simulink model "eCS_Algo_Simulation_2015b_opti - original"  (R2015b)
settings: Solver=ode1  StartTime=0.0  StopTime=3  FixedStep=1/80000  RelTol=1e-3
PreLoadFcn:
  | if exist('tl_preloadfcn','file'), tl_preloadfcn(gcs,402); end
PostLoadFcn:
  | , if any(exist('dsrtsu_mdlpostloadfcn', 'file') == [2, 3, 6]), try dsrtsu_mdlpostloadfcn('Execute', bdroot); catch fprintf('Error in PostLoadFcn (dsrtsu_mdlpostloadfcn) for model "%s":\n %s\n', bdroot, lasterr); end, end,
  | if exist('tl_postloadfcn','file'), tl_postloadfcn(gcs,402); end
InitFcn:
  | Omegan=1.3024e+03;
  | xi=0.9; %0.48
  | K=0.1931;
  | K1=0.0198;
  | TauLocked=0.00255;
  | TauUnLocked=0.0042;
  | Kp=1/(2*K1);
  | Ki=Kp/((TauLocked+TauUnLocked)/2);
  | if exist('tlds_init','file'), tlds_init(gcs); end
StartFcn:
  | if exist('tlds_start','file'), tlds_start(gcs); end
StopFcn:
  | if exist('tlds_stop','file'), tlds_stop(gcs); end
model workspace (MAT data in the model file):
  au8PrevExecProfile = [0 0 0 0 0 0]
values from neighbouring files (symbols this model uses):
  AccSensor = 5    [Parameter_eCS_Algo.m]
  AlgoType = 0    [Parameter_eCS_Algo.m]
  Cxy = 1*0.017    (= 0.017)    [Acc_Init_SelV1.m]
  Cxz = 1*0.017    (= 0.017)    [Acc_Init_SelV1.m]
  Cyx = 1*0.017    (= 0.017)    [Acc_Init_SelV1.m]
  Cyz = 1*0.017    (= 0.017)    [Acc_Init_SelV1.m]
  Czx = 1*0.017    (= 0.017)    [Acc_Init_SelV1.m]
  Czy = 1*0.017    (= 0.017)    [Acc_Init_SelV1.m]
  Forced_Oscillation = 0    [Parameter_eCS_Algo.m]    (also in run_Rotation_sim.m = run)
  FreqTemperature = 10    [Acc_Init_SelV1.m]
  MaxSensorOffset = 0.3    [Acc_Init_SelV1.m]
  Mean_x_noise = 4e-3    (= 0.004)    [Acc_Init_SelV1.m]
  Mean_y_noise = 4e-3    (= 0.004)    [Acc_Init_SelV1.m]
  Mean_z_noise = 4e-3    (= 0.004)    [Acc_Init_SelV1.m]
  ODR = 8000    [Acc_Init_SelV1.m]
  offsetcorrection_on_off = 0    [Parameter_eCS_Algo.m]
  phi_pulse_rotation = 0    [Parameter_eCS_Algo.m]    (also in run_Rotation_sim.m = angle)
  pulsetype = 2    [Parameter_eCS_Algo.m]    (also in run_simulation.m = j; run_simulation_ActiveX.m = j)
  Range = 4    [Acc_Init_SelV1.m]
  sensitivity_optimisation = 0    [Parameter_eCS_Algo.m]
  TempBias = 0    [Acc_Init_SelV1.m]
  TemperatureAmp = 0    [Acc_Init_SelV1.m]
  Var_x_noise = 1.84e-9    (= 1.84e-09)    [Acc_Init_SelV1.m]
  Var_y_noise = 2.025e-09    [Acc_Init_SelV1.m]
  Var_z_noise = 1.374e-09    [Acc_Init_SelV1.m]
  w_x = 2*pi*F_x    (= 376.991118431)    [Acc_Init_SelV1.m]
  w_y = 2*pi*F_y    (= 376.991118431)    [Acc_Init_SelV1.m]
  w_z = 2*pi*F_z    (= 376.991118431)    [Acc_Init_SelV1.m]
  x_max_temp_drift = 0.061    [Acc_Init_SelV1.m]
  x_offset_enable = 0    [Acc_Init_SelV1.m]
  x_run_to_run_drift = 0.0    (= 0)    [Acc_Init_SelV1.m]
  x_temp_co_drift = 0.000    (= 0)    [Acc_Init_SelV1.m]
  Xi_x = 0.7    [Acc_Init_SelV1.m]
  Xi_y = 0.7    [Acc_Init_SelV1.m]
  Xi_z = 0.7    [Acc_Init_SelV1.m]
  y_max_temp_drift = 0.061    [Acc_Init_SelV1.m]
  y_offset_enable = 0    [Acc_Init_SelV1.m]
  y_run_to_run_drift = 0.0    (= 0)    [Acc_Init_SelV1.m]
  y_temp_co_drift = 0.000    (= 0)    [Acc_Init_SelV1.m]
  z_max_temp_drift = 0.13    [Acc_Init_SelV1.m]
  z_offset_enable = 0    [Acc_Init_SelV1.m]
  z_run_to_run_drift = 0.0    (= 0)    [Acc_Init_SelV1.m]
  z_temp_co_drift = 0.000    (= 0)    [Acc_Init_SelV1.m]
undefined symbols (not defined in the file or in its folder): ddv, DiscIntNeverNeededParam, gmw_roada_x__m_s__, gmw_roada_y__m_s__, gmw_roadtime_2kHz, KSF_50_a_x, KSF_50_a_y, KSF_50_time, KSG_30_a_x, KSG_30_a_y, KSG_30_time, Meldorf_HindenburgstraAcceleration_x__m_s_2_, Meldorf_HindenburgstraAcceleration_y__m_s_2_, Meldorf_HindenburgstraAcceleration_z__m_s_2_, Meldorf_HindenburgstraTime__s_, pulse_FF27, pulse_MPDB, pulse_ODB40, pulse_ODB64, pulse_USNCAP, pulsetime_FF27, pulsetime_MPDB, pulsetime_ODB40, pulsetime_ODB64, pulsetime_USNCAP, Rauasphalt_60_a_x, Rauasphalt_60_a_y, Rauasphalt_60_time, sigbuilder_block, VW_416_2kHza_x_2kHz, VW_416_2kHza_y_2kHz, VW_416_2kHztime_2kHz
libraries: simulink x20, tllib x16, tl_autosar_lib x12, simulink_extras x7, LIB_TF_G_12_StepControl x2, LIB_TF_G_111 x1, LIB_TF_G_112 x1
(part 1 of 9)
PreSaveFcn:
  | if exist('tl_presavefcn','file'), tl_presavefcn(gcs); end
CloseFcn:
  | if exist('tl_closefcn','file'), tl_closefcn(gcs); end
settings Model: Tag=struct('sfcnName','Subsystem_sf','subFunction','','srcSubsystem','')  DSRTSU_INTERNAL_RTI_VER=520  DSRTSU_INTERNAL_RTI_TYPE=rti1103  DSRTSU_INTERNAL_RTIFPGA=110  RTICANMMDATA=struct('GeneralSetupData',struct('modelroot','P:\ES\USER\Hinrichs\Projekte\93D48_eCS\Simulink\20200514_eCS_Simulation_package','generalsettings',struct('filesettings',struct('destfolder',struct('Name','RTICANMM_FILES','Check',1),'buildfolder',struct('Name','.','Check',1),'AbsDestfolder',struct('Name','P:\ES\USER\Hinrichs\Projekte\93D48_eCS\Simulink\20200514_eCS_Simulation_package\RTICANMM_FILES'),'AbsBuildfolder',struct('Name','P:\ES\USER\Hinrichs\Projekte\93D48_eCS\Simulink\20200514_eCS_Simulation_package'))),'options',struct('addpaths',1,'rmpaths',1,'addtrcexclusion',logical(1),'cannavigator',struct('checkmonitoring',0),'show_usrtrc',0,'use_usrtrc',0),'advanced',struct('options',[1 1 1 1 1 1 1 1 1 1 1 1 1 1 1 1 1 1 1 1 1 1 1 1 1 1 1 1 1 1 1 1 1 1 1 1 1 1 1 1 1 1 1 1 1 1 1 1 1 1 1 1 1 1 1 1 1 1 1 1 1 1 1 1 1 1 1 1 1 1 1 1 1 1 1 1 1 1 1 1 1 1 1 1 1 1 1 1 1 1 1 1 1 1 1 1 1 1 1 1]),'MPSetup',{{}},'modelname','eCS_Algo_Simulation','block','eCS_Algo_Simulation'))  DSRTSU_INTERNAL_RTIFLEXRAYCONFIG=110  TL_MAIN_DATA={'date',739018.44784596062,'advcodeopt',{'IgnoreAccessFunctionsInOwnModule';'on';'OptimizationIterationThreshold';100;'SideEffectFreeAnalysisThreshold';1000000;'ReuseStructHandling';1;'ReplaceUnrolledVectorsAndMatricesByScalars';'on';'GlobalOptimizationIterationThreshold';100;'ForceBooleanOperandsInBooleanOperations';'off'},'codegenerationmode',2}  TLRevision=402  DS_PROJECTFILE=eCS_DD.dd  Creator=heiko.hinrichs  LastModifiedBy=victor.popina
settings SolverCC: AutoInsertRateTranBlk=on
settings DataIOCC: SaveFormat=Array
settings OptimizationCC: BlockReduction=off  OptimizeBlockIOStorage=off  BufferReuse=off  GlobalBufferReuse=off  ExpressionFolding=off  ExpressionDepthLimit=2147483647  LocalBlockOutputs=off
settings DebuggingCC: UnderspecifiedInitializationDetection=Classic  MergeDetectMultiDrivingBlocksExec=none  SolverPrmCheckMsg=warning  FcnCallInpInsideContextMsg=EnableAllAsWarning  BusObjectLabelMismatch=error  AllowSymbolicDim=on  StateNameClashWarn=warning  StrictBusMsg=ErrorOnBusTreatedAsVector  NonBusSignalsTreatedAsBus=error
settings HardwareCC: ProdBitPerPointer=32  ProdLargestAtomicInteger=Integer  ProdEndianess=BigEndian  ProdWordSize=32  ProdHWDeviceType=Custom Processor->Custom  TargetHWDeviceType=Custom Processor->Custom
settings RTWCC: SystemTargetFile=rti1103.tlc  MakeCommand=make_rti  TemplateMakefile=rti1103.tmf  Description=dSPACE DS1103 Hardware Platform
settings STFCustomTargetCC: ParMdlRefBuildCompliant=on  ConcurrentExecutionCompliant=off  GeneratePreprocessorConditionals=Use local settings  CPPClassGenCompliant=off  GRTInterface=off  SystemTargetFile=rti1103.tlc
settings GRTTargetCC: CompOptLevelCompliant=off  ConcurrentExecutionCompliant=off  CombineOutputUpdateFcns=off  MatFileLogging=off  CPPClassGenCompliant=off  UseToolchainInfoCompliant=off  ExtModeMexFile=noextcomm
settings ConfigComp: CovModelRefEnable=Off

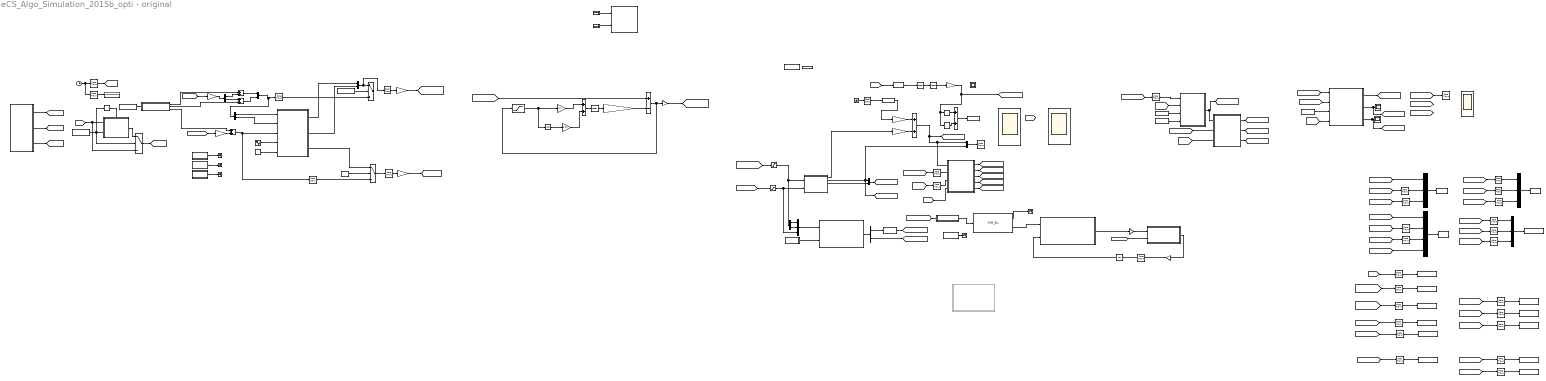
== system eCS_Algo_Simulation_2015b_opti - original ==
  note: ECS
  note: [-39.22 ; 39.22] m/s²
      | [-4 ; 4] g
  note: "retractor locked"
  note: Outputs
  note: Retractor mechanics
  note: Solenoid
  note: Offset correction
  note: Input pulses / load cases
  note: Sensor model Ziad
  note: "lever locked" (solenoid locked)
  note: "lock decision" (algo "locked")
  A_to_mA : Gain  Gain=1000
  Accelerometer : Subsystem
  Add{,1,3..5,7} (6 alike) : Sum
  Add2 : Sum  Inputs=+-
  Bus Selector1 : BusSelector  OutputSignals=b8EcsFlag,u16BallPosition
  BusCreator : BusCreator  Inputs=3
  Clock : Clock
  Compare To Constant : simulink/Logic and Bit Operations/Compare To Constant  relop=>=  const=25  OutDataTypeStr=uint8
  Compare To Constant1 : simulink/Logic and Bit Operations/Compare To Constant  relop=>=  const=50  OutDataTypeStr=uint8
  Compare To Constant4 : simulink/Logic and Bit Operations/Compare To Constant  relop=~=  const=0  OutDataTypeStr=boolean
  Constant : Constant  Value=0
  Constant2 : Constant  Value=Forced_Oscillation
  Crash signal1 : Subsystem  Tag=STV Subsys  LoadFcn=sigbuilder_block('load');  StartFcn=sigbuilder_block('start');  StopFcn=sigbuilder_block('stop');  ClipboardFcn=sigbuilder_block('clipboard');  mask(Sigbuilder block){}
      mask help: Simulink:masks:SigbuilderBlock_MD
      mask init:
      | if ~strcmp(get_param(bdroot(gcbh),'SimulationStatus'),'stopped') tuvar = sigbuilder_block('maskInit'); end
      settings: CopyFcn=sigbuilder_block('copy');  DeleteFcn=sigbuilder_block('delete');  ModelCloseFcn=sigbuilder_block('modelClose');  PreSaveFcn=sigbuilder_block('preSave');  PauseFcn=sigbuilder_block('pause');  ContinueFcn=sigbuilder_block('continue');  NameChangeFcn=sigbuilder_block('namechange');  OpenFcn=sigbuilder_block('open',[95.25 97.5 1200 576 ]);  CloseFcn=sigbuilder_block('close');
      mask Display: plot(0, 0, 100, 100,[2, 2, 32, 32, 2], [68, 8, 8, 68, 68],[32, 2], [38, 38], [32, 19, 2],[53, 60, 44], [32, 17, 17, 2],[16, 16, 31, 31]);txt = getActiveGroup(gcbh);text(2, 100, txt,'verticalAlignment', 'top');
  Crash signal3 : Subsystem  Tag=STV Subsys  LoadFcn=sigbuilder_block('load');  StartFcn=sigbuilder_block('start');  StopFcn=sigbuilder_block('stop');  ClipboardFcn=sigbuilder_block('clipboard');  mask(Sigbuilder block){}
      mask help: Simulink:masks:SigbuilderBlock_MD
      mask init:
      | if ~strcmp(get_param(bdroot(gcbh),'SimulationStatus'),'stopped') tuvar = sigbuilder_block('maskInit'); end
      settings: CopyFcn=sigbuilder_block('copy');  DeleteFcn=sigbuilder_block('delete');  ModelCloseFcn=sigbuilder_block('modelClose');  PreSaveFcn=sigbuilder_block('preSave');  PauseFcn=sigbuilder_block('pause');  ContinueFcn=sigbuilder_block('continue');  NameChangeFcn=sigbuilder_block('namechange');  OpenFcn=sigbuilder_block('open',[54 1.5 1200 540 ]);  CloseFcn=sigbuilder_block('close');
      mask Display: plot(0, 0, 100, 100,[2, 2, 32, 32, 2], [68, 8, 8, 68, 68],[32, 2], [38, 38], [32, 19, 2],[53, 60, 44], [32, 17, 17, 2],[16, 16, 31, 31]);txt = getActiveGroup(gcbh);text(2, 100, txt,'verticalAlignment', 'top');
  Data Type Conversion : DataTypeConversion
  Demux : Demux  Outputs=2
  Demux2 : Demux  Outputs=2
  Demux3 : Demux  Outputs=2
  Discrete-Time Integrator : DiscreteIntegrator  InitialConditionSetting=State (most efficient)  SampleTime=-1  ICPrevOutput=DiscIntNeverNeededParam  ICPrevScaledInput=DiscIntNeverNeededParam
  Discrete-Time Integrator1 : DiscreteIntegrator  InitialConditionSetting=State (most efficient)  SampleTime=-1  ICPrevOutput=DiscIntNeverNeededParam  ICPrevScaledInput=DiscIntNeverNeededParam
  Discrete-Time Integrator4 : DiscreteIntegrator  gainval=1  InitialConditionSetting=State (most efficient)  SampleTime=-1  LimitOutput=on  UpperSaturationLimit=0.3 * 9.81  LowerSaturationLimit=-0.3 * 9.81  ICPrevOutput=DiscIntNeverNeededParam  ICPrevScaledInput=DiscIntNeverNeededParam
  FSM : Subsystem  Tag=TargetLink Simulation Frame  Commented=on  mask(TL_SimFrame){}
      settings: CopyFcn=if exist('tl_copyfcn','file'), tl_copyfcn(gcbh); end  NameChangeFcn=if exist('tl_framenamechangefcn','file'), tl_framenamechangefcn(gcbh); end
      settings: OpenFcn=|
      | if exist('open_tlsubsystem','file')
      |    open_tlsubsystem(gcbh);
      | else
      |    tlsubsystem = ...
      |       find_system(gcb, ...
      |       'LookUnderMasks','on', ...
      |       'FollowLinks','on', ...
      |       'Tag','MIL Subsystem');
      |    open_system(tlsubsystem);
      | end
      mask Display: disp('TargetLink\nModel-\nin-the-loop\nmode')
  FSM_prrEcsAlgoFlag : Subsystem
  FSM_prrVehicleInputs : Subsystem
  G-lock Scope new : Scope  NumInputPorts=4
  Gain : Gain  Gain=AlgoType
  Gain1 : Gain  Gain=1- AlgoType
  Ground : Ground
  Input (Pulse/ Angle)1 : Subsystem
  MIL Handler : tllib/MIL Handler  data={'date',730486}
  Mux : Mux  Inputs=3
  Mux{1,3,8,10} (4 alike) : Mux  Inputs=2
  Mux2 : Mux
  Mux4 : Mux  Inputs=3
  Mux9 : Mux  Inputs=3
  Noisy : Subsystem  Tag=STV Subsys  LoadFcn=sigbuilder_block('load');  StartFcn=sigbuilder_block('start');  StopFcn=sigbuilder_block('stop');  ClipboardFcn=sigbuilder_block('clipboard');  mask(Sigbuilder block){}
      mask help: Simulink:masks:SigbuilderBlock_MD
      mask init:
      | if ~strcmp(get_param(bdroot(gcbh),'SimulationStatus'),'stopped') tuvar = sigbuilder_block('maskInit'); end
      settings: CopyFcn=sigbuilder_block('copy');  DeleteFcn=sigbuilder_block('delete');  ModelCloseFcn=sigbuilder_block('modelClose');  PreSaveFcn=sigbuilder_block('preSave');  PauseFcn=sigbuilder_block('pause');  ContinueFcn=sigbuilder_block('continue');  NameChangeFcn=sigbuilder_block('namechange');  OpenFcn=sigbuilder_block('open',[54 1.5 1200 535.5 ]);  CloseFcn=sigbuilder_block('close');
      mask Display: plot(0, 0, 100, 100,[2, 2, 32, 32, 2], [68, 8, 8, 68, 68],[32, 2], [38, 38], [32, 19, 2],[53, 60, 44], [32, 17, 17, 2],[16, 16, 31, 31]);txt = getActiveGroup(gcbh);text(2, 100, txt,'verticalAlignment', 'top');
  PWM_to_V : Gain  Gain=14/32768
  PrevSolenoidCurrent : UnitDelay  SampleTime=-1
  Pulse measured1 : RateTransition  Deterministic=off  OutPortSampleTime=1/2000
  Pulse measured2 : RateTransition
  Pulse measured3 : RateTransition  Deterministic=off  OutPortSampleTime=1/2000
  Pulse measured4 : RateTransition
  Pulse raw (g) : Gain  Gain=1/9.807
  Pulse raw (g)1 : Gain  Gain=1/9.807
  Pulse raw1 : Gain  Gain=9.807
  Pulse raw2 : Gain  Gain=9.807
  Pulse with Offsetcorr. : Gain
  Rate Transition{,1..2,4..6,9..11,15,22} (11 alike) : RateTransition
  Rate Transition{12..14,16..21} (9 alike) : RateTransition  OutPortSampleTime=1/10000
  Rate Transition{3,7,23..24,26..27,30..32} (9 alike) : RateTransition  OutPortSampleTime=1/2000
  Rate Transition25 : RateTransition  OutPortSampleTime=1/5
  S-Function Builder : S-Function  InitFcn=try, set_param(gcb,'FunctionName','FSM_SIL'), end  FunctionName=FSM_SIL  SFunctionModules=FSM_SIL_wrapper  SFunctionDeploymentMode=off  EnableBusSupport=off  mask(S-Function Builder){}
      mask help: Simulink:masks:SFunctionBuilder_MD
      mask init:
      | val = [[.9  0.75 0.75 1 1 .9 .9 1]',[1 1 0.75 0.75 .9 .9 1 .9]'];try , sys = get_param(gcb,'SfunBuilderFcnName');if isempty(sys), sys = get_param(gcb,'FunctionName'); end,catch, sys = get_param(gcb,'FunctionName'); end
      settings: CopyFcn=set_param(gcbh,'LinkStatus','none')  PreSaveFcn=try, set_param(gcb,'FunctionName','FSM_SIL'), end  OpenFcn=sfunctionwizard(gcbh)
      mask Display: plot(val(:,1),val(:,2)),disp(sys), port_label('input',1,'prrEcsAlgoFlag'), port_label('output',1,'psrSolenoidState'), port_label('output',2,'psrFsmProfile')
  SAD : Subsystem  Tag=TargetLink Simulation Frame  mask(TL_SimFrame){}
      settings: CopyFcn=if exist('tl_copyfcn','file'), tl_copyfcn(gcbh); end  NameChangeFcn=if exist('tl_framenamechangefcn','file'), tl_framenamechangefcn(gcbh); end
      settings: OpenFcn=|
      | if exist('open_tlsubsystem','file')
      |    open_tlsubsystem(gcbh);
      | else
      |    tlsubsystem = ...
      |       find_system(gcb, ...
      |       'LookUnderMasks','on', ...
      |       'FollowLinks','on', ...
      |       'Tag','MIL Subsystem');
      |    open_system(tlsubsystem);
      | end
      mask Display: disp('TargetLink\nModel-\nin-the-loop\nmode')
  Saturation : Saturate  UpperLimit=+39.3  LowerLimit=-39.3
  "Saturation acc. script, i.e.+-0,3g (max. offset of sensor after ageing)" : Saturate  UpperLimit=MaxSensorOffset * 9.807  LowerLimit=-MaxSensorOffset * 9.807
  Saturation1 : Saturate  UpperLimit=+39.22  LowerLimit=-39.22
  Scope1 : Scope  NumInputPorts=3
  Sign : Signum
  Solenoid Model : Subsystem  TreatAsAtomicUnit=on
  Subsystem : Subsystem  Tag=MIL Subsystem  Description=a  mask(MIL Subsystem){}
      settings: CopyFcn=if exist('tl_copyfcn','file'), tl_copyfcn(gcbh); end  NameChangeFcn=if exist('tl_namechangefcn','file'), tl_namechangefcn(gcbh); end  DestroyFcn=if exist('update_tl_main_dlg','file'), update_tl_main_dlg('TL_subs_display'); end
      mask Display: disp('TargetLink Subsystem')
  Switch : Switch  Criteria=u2 ~= 0
  TargetLink Main Dialog : tllib/TargetLink Main Dialog  data=[]
  Temperature : Sin  Amplitude=TemperatureAmp  Bias=TempBias  Frequency=FreqTemperature  SampleTime=0
  Terminator{,1..4} (5 alike) : Terminator
  Tilt_Lock_Scop1 : Scope  NumInputPorts=2
  To Workspace : ToWorkspace  VariableName=triggers_s  SaveFormat=Timeseries  SampleTime=-1
      settings: MaxDataPoints=1  Save2DSignal=2-D array (concatenate along first dimension)
  To Workspace1 : ToWorkspace  VariableName=pulse  SaveFormat=Timeseries  SampleTime=-1
      settings: Save2DSignal=2-D array (concatenate along first dimension)
  To Workspace10 : ToWorkspace  VariableName=time  SampleTime=-1
      settings: Save2DSignal=2-D array (concatenate along first dimension)
  To Workspace11 : ToWorkspace  VariableName=trigger_eCS_REF  SampleTime=-1
      settings: Save2DSignal=2-D array (concatenate along first dimension)
  To Workspace14 : ToWorkspace  VariableName=s_ball_REF  SampleTime=-1
      settings: Save2DSignal=2-D array (concatenate along first dimension)
  To Workspace15 : ToWorkspace  VariableName=ball_a2  SampleTime=-1
      settings: Save2DSignal=2-D array (concatenate along first dimension)
  To Workspace16 : ToWorkspace  VariableName=trigg_a2  SampleTime=-1
      settings: Save2DSignal=2-D array (concatenate along first dimension)
  To Workspace2 : ToWorkspace  VariableName=pulse_sensor_output  SaveFormat=Timeseries  SampleTime=-1
      settings: Save2DSignal=2-D array (concatenate along first dimension)
  To Workspace3 : ToWorkspace  VariableName=pulse_with_offsetcorrection  SaveFormat=Timeseries  SampleTime=-1
      settings: Save2DSignal=2-D array (concatenate along first dimension)
  To Workspace4 : ToWorkspace  VariableName=s_ball  SaveFormat=Timeseries  SampleTime=-1
      settings: Save2DSignal=2-D array (concatenate along first dimension)
  To Workspace5 : ToWorkspace  VariableName=trigger_eCS  SaveFormat=Timeseries  SampleTime=-1
      settings: Save2DSignal=2-D array (concatenate along first dimension)
  To Workspace6 : ToWorkspace  VariableName=triggers_times  SampleTime=-1
      settings: MaxDataPoints=1  Save2DSignal=2-D array (concatenate along first dimension)
  To Workspace7 : ToWorkspace  VariableName=s_rig  SaveFormat=Timeseries  SampleTime=-1
      settings: Save2DSignal=2-D array (concatenate along first dimension)
  To Workspace8 : ToWorkspace  VariableName=s_locking  SaveFormat=Timeseries  SampleTime=-1
      settings: Save2DSignal=2-D array (concatenate along first dimension)
  To Workspace9 : ToWorkspace  VariableName=triggercounts  SampleTime=-1
      settings: Save2DSignal=2-D array (concatenate along first dimension)
  Vektor_addition_Pulse1 : Fcn  Expr=sqrt( (u(1)*u(1)) + (u(2)*u(2)) )
  acc. measurement direct/via acc. sensor : Switch  Criteria=u2 > Threshold
  acc. measurement direct/via acc. sensor1 : Switch  Criteria=u2 > Threshold
  "acc. sensor type: 0=direct, 1=AD, 2=ST, 3=TDK, 4=NXP" : Constant  Value=AccSensor  VectorParams1D=off
  "acc. sensor type: 0=direct, 1=AD, 2=ST, 3=TDK, 4=NXP1" : Constant  Value=AccSensor  VectorParams1D=off
  delta-t to lock (ms) : Constant  Value=5
  delta-t to unlock (ms) : Constant  Value=7
  deviation dependent correction: 0.1/s ~10mg/s at 1m/s²deviation ~0,6°/s with saturation +-0,3g: max. 30mg/s / ~1,8°/s possible : Gain  Gain=0.1
  eCS : Subsystem  Tag=TargetLink Simulation Frame  mask(TL_SimFrame){}
      settings: CopyFcn=if exist('tl_copyfcn','file'), tl_copyfcn(gcbh); end  NameChangeFcn=if exist('tl_framenamechangefcn','file'), tl_framenamechangefcn(gcbh); end
      settings: OpenFcn=|
      | if exist('open_tlsubsystem','file')
      |    open_tlsubsystem(gcbh);
      | else
      |    tlsubsystem = ...
      |       find_system(gcb, ...
      |       'LookUnderMasks','on', ...
      |       'FollowLinks','on', ...
      |       'Tag','MIL Subsystem');
      |    open_system(tlsubsystem);
      | end
      mask Display: disp('TargetLink\nModel-\nin-the-loop\nmode')
  eCS Algo new2 : Subsystem
  eCS_prrAccelMtrPerSecSqd_stAccelMtrPerSecSqd : Subsystem
  eCS_prrEcsDiagRequest : Subsystem
  eCS_prrEcsDiagRequest_b8DiagReq1 : Subsystem
  locking distance (mm) : Constant  Value=18.13
  offset correction on/off : Gain  Gain=offsetcorrection_on_off  OutMin=[0]  OutMax=[1]
  oscilliation generator : Subsystem
  permanent correction: 0.01m/s²/s ~1mg/s ~0,06°/s : Gain  Gain=0.01
  phi-pulse-rotation (°) : Constant  Value=phi_pulse_rotation
  pulse rotation around z-axis : Subsystem
  retractor locking trigger : MATLAB Function  TreatAsAtomicUnit=on
  s-locking retractor (mm) : Scope
  s-rig (mm) new : Scope
  s-rig-trigger new : DataTypeConversion
  s-rig-trigger new1 : DataTypeConversion
  s_rig in mm : Gain  Gain=1000
  solenoid time delay : MATLAB Function  TreatAsAtomicUnit=on
  time (0.2s-steps) : Display
  "trigger travels, times and counts" : MATLAB Function  TreatAsAtomicUnit=on
  "trigger travels, times and counts1" : MATLAB Function  TreatAsAtomicUnit=on
  triggertime_retractor (ms) : Scope
  wires:
  Discrete-Time Integrator1/1 -> s_rig in mm/1
  Discrete-Time Integrator/1 -> Discrete-Time Integrator1/1
  Add4/1 -> "trigger travels, times and counts"/1(trigger), Mux3/1, [trigger_eCS]
  s_rig in mm/1 -> [s], Compare To Constant/1, Compare To Constant1/1
  Compare To Constant/1 -> Add/2
  Compare To Constant1/1 -> Add/1
  Add/1 -> s-rig-trigger new/1
  Mux3/1 -> Rate Transition4/1
  "Saturation acc. script, i.e.+-0,3g (max. offset of sensor after ageing)"/1 -> Sign/1, deviation dependent correction: 0.1/s ~10mg/s at 1m/s²deviation ~0,6°/s with saturation +-0,3g: max. 30mg/s / ~1,8°/s possible/1
  Sign/1 -> permanent correction: 0.01m/s²/s ~1mg/s ~0,06°/s/1
  offset correction on/off/1 -> Add2/2
  Discrete-Time Integrator4/1 -> offset correction on/off/1
  Add3/1 -> Discrete-Time Integrator4/1
  deviation dependent correction: 0.1/s ~10mg/s at 1m/s²deviation ~0,6°/s with saturation +-0,3g: max. 30mg/s / ~1,8°/s possible/1 -> Add3/1
  permanent correction: 0.01m/s²/s ~1mg/s ~0,06°/s/1 -> Add3/2
  Add2/1 -> Pulse with Offsetcorr./1, "Saturation acc. script, i.e.+-0,3g (max. offset of sensor after ageing)"/1
  Clock/1 -> Rate Transition25/1, Rate Transition2/1
  [time] -> solenoid time delay/2(time)
  [trigger_eCS] -> Rate Transition/1
  solenoid time delay/1(trigger_out) -> "trigger travels, times and counts1"/1(trigger), [locking_solenoid]
  [trigger_eCS] -> Rate Transition1/1
  Temperature/1 -> Accelerometer/4(Temperature)
  Constant/1 -> Accelerometer/5(Max temp. drift)
  Accelerometer/2(Out Y) -> Mux8/2  "sensor_ay"
  Accelerometer/1(Out X) -> Mux8/1  "sensor_ax"
  Demux2/2 -> Accelerometer/2(In Y)
  Crash signal1/1(Signal 1) -> Terminator/1
  Demux2/1 -> Accelerometer/1(In X)
  Pulse with Offsetcorr./1 -> [Pulse_with_offsetcorrection]
  locking distance (mm)/1 -> retractor locking trigger/3(s_mech_locking)
  [time] -> retractor locking trigger/4(time)
  [s] -> retractor locking trigger/2(s)
  [locking_solenoid] -> retractor locking trigger/1(trigger_solenoid)
  retractor locking trigger/1(trigger_retractor) -> [locking_retractor]
  retractor locking trigger/2(triggertime_retractor) -> [triggertime_retractor], triggertime_retractor (ms)/1
  retractor locking trigger/3(s_locking) -> [s_locking_retractor], s-locking retractor (mm)/1
  [Pulse] -> Vektor_addition_Pulse1/1
  Vektor_addition_Pulse1/1 -> Discrete-Time Integrator/1
  [Pulse_no_offsetcorrection] -> Add2/1
  Noisy/1(Signal 1) -> Terminator2/1
  Crash signal3/1(Signal 1) -> Terminator3/1
  Rate Transition/1 -> solenoid time delay/1(trigger)
  Mux/1 -> To Workspace/1
  Rate Transition2/1 -> [time]
  [time] -> Rate Transition5/1
  Rate Transition5/1 -> "trigger travels, times and counts"/3(time)
  "trigger travels, times and counts"/2(triggertime) -> [triggertime_eCS]
  [s_locking_retractor] -> Rate Transition6/1
  Rate Transition6/1 -> Mux/3
  [triggertime_eCS] -> Mux2/1
  [triggertime_solenoid] -> Rate Transition9/1
  Rate Transition9/1 -> Mux2/2
  [triggertime_retractor] -> Rate Transition10/1
  Rate Transition10/1 -> Mux2/3
  "trigger travels, times and counts"/1(s_locking) -> [s_locking_eCS]
  [s] -> Rate Transition11/1
  Rate Transition11/1 -> "trigger travels, times and counts"/2(s)
  [s_locking_eCS] -> Mux/1
  [s] -> "trigger travels, times and counts1"/2(s)
  [time] -> "trigger travels, times and counts1"/3(time)
  "trigger travels, times and counts1"/2(triggertime) -> [triggertime_solenoid]
  "trigger travels, times and counts1"/1(s_locking) -> [s_locking_solenoid]
  [s_locking_solenoid] -> Rate Transition15/1
  Rate Transition15/1 -> Mux/2
  delta-t to unlock (ms)/1 -> solenoid time delay/4(dt_to_unlock)
  delta-t to lock (ms)/1 -> solenoid time delay/3(dt_to_lock)
  Mux8/1 -> Pulse measured1/1, acc. measurement direct/via acc. sensor/1
  "acc. sensor type: 0=direct, 1=AD, 2=ST, 3=TDK, 4=NXP"/1 -> acc. measurement direct/via acc. sensor/2
  Pulse measured2/1 -> acc. measurement direct/via acc. sensor/3
  [Pulse] -> Rate Transition16/1
  Rate Transition16/1 -> To Workspace1/1
  Rate Transition17/1 -> To Workspace2/1
  [Pulse_no_offsetcorrection] -> Rate Transition17/1
  Rate Transition18/1 -> To Workspace3/1
  [Pulse_with_offsetcorrection] -> Rate Transition18/1
  Rate Transition19/1 -> To Workspace4/1
  [s_ball] -> Rate Transition19/1
  Rate Transition20/1 -> To Workspace5/1
  Mux2/1 -> To Workspace6/1
  Rate Transition13/1 -> To Workspace7/1
  [s] -> Rate Transition13/1
  Rate Transition12/1 -> Mux4/2
  [s_locking_solenoid] -> Rate Transition12/1
  [s_locking_eCS] -> Rate Transition21/1
  Rate Transition14/1 -> Mux4/3
  [s_locking_retractor] -> Rate Transition14/1
  Mux4/1 -> To Workspace8/1
  Rate Transition21/1 -> Mux4/1
  [Pulse_with_offsetcorrection] -> Saturation/1
  Rate Transition22/1 -> s-rig-trigger new1/1
  s-rig-trigger new1/1 -> Gain/1
  Gain/1 -> Add4/1
  Gain1/1 -> Add4/2
  "trigger travels, times and counts"/3(triggercounts) -> [triggercounts_eCS]
  "trigger travels, times and counts1"/3(triggercounts) -> [triggercounts_solenoid]
  [triggercounts_solenoid] -> Rate Transition24/1
  [triggercounts_eCS] -> Rate Transition23/1
  Rate Transition23/1 -> Mux9/1
  Rate Transition24/1 -> Mux9/2
  Rate Transition25/1 -> time (0.2s-steps)/1
  [time] -> Rate Transition26/1
  Rate Transition26/1 -> To Workspace10/1
  [trigger_eCS] -> Rate Transition20/1
  Rate Transition27/1 -> To Workspace11/1
  Rate Transition30/1 -> To Workspace14/1
  [trigger_eCS] -> Rate Transition27/1
  [s_ball_only] -> Rate Transition30/1
  Saturation/1 -> Demux/1, eCS Algo new2/1(Pulse X,Y)
  [Trigg_a2] -> Rate Transition32/1
  [Ball_a2] -> Rate Transition31/1
  Rate Transition31/1 -> To Workspace15/1
  Rate Transition32/1 -> To Workspace16/1
  Pulse measured1/1 -> Pulse raw1/1
  Pulse raw1/1 -> [Pulse_no_offsetcorrection]
  [Pulse_rotated] -> Pulse raw (g)/1
  Input (Pulse/ Angle)1/1("Pulse_profile ") -> [Pulse]  "pulse X,Y in m/s²"
  Input (Pulse/ Angle)1/3(angle in °) -> [angle]
  [Pulse] -> Switch/3, pulse rotation around z-axis/1(pulse in m/s²)
  phi-pulse-rotation (°)/1 -> Switch/2, Compare To Constant4/1, pulse rotation around z-axis/2(rotation angle)
  Compare To Constant4/1 -> pulse rotation around z-axis/Enable
  pulse rotation around z-axis/1(pulse rotated in m/s²) -> Switch/1
  Input (Pulse/ Angle)1/2(Pulse z-axis) -> [Pulse_z_axis]  "pulse Z in m/s²"
  [Pulse_z_axis] -> Pulse raw (g)1/1
  Accelerometer/3(Out Z) -> acc. measurement direct/via acc. sensor1/1  "sensor_az"
  Pulse measured3/1 -> Pulse raw2/1
  "acc. sensor type: 0=direct, 1=AD, 2=ST, 3=TDK, 4=NXP1"/1 -> acc. measurement direct/via acc. sensor1/2
  Pulse raw2/1 -> [Pulse_z_axis_sensor]
  Pulse measured4/1 -> acc. measurement direct/via acc. sensor1/3
  eCS Algo new2/2(s_ball) -> [s_ball_only], Mux10/1, Mux3/2  "pBall_Simulink"
  eCS Algo new2/1(Trigger eCS) -> Gain1/1
  eCS Algo new2/3(s_ball_x- + y-components) -> Mux10/2
  [Pulse_z_axis_sensor] -> Saturation1/1
  Mux10/1 -> [s_ball]
  [Trigg_a2] -> "trigger travels, times and counts"/4(eCSTrigger)
  "trigger travels, times and counts"/4(triggerCountsTL) -> [triggercounts_TL]
  Mux9/1 -> To Workspace9/1
  [triggercounts_TL] -> Rate Transition3/1
  Rate Transition3/1 -> Mux9/3
  "trigger travels, times and counts"/5(triggerTimeTL) -> [triggerTme_TL]
  [triggerTme_TL] -> Mux2/4
  acc. measurement direct/via acc. sensor1/1 -> Pulse measured3/1
  Switch/1 -> [Pulse_rotated]
  Mux1/1 -> Demux2/1, Pulse measured2/1
  Pulse raw (g)/1 -> Demux3/1
  Pulse raw (g)1/1 -> Add5/2
  Add5/1 -> Accelerometer/3(In Z), Pulse measured4/1
  Demux3/2 -> Add7/1
  Demux3/1 -> Add1/2
  Add1/1 -> Mux1/1
  Add7/1 -> Mux1/2
  Constant2/1 -> oscilliation generator/1(bOscillationReq)
  oscilliation generator/1(Oscillation_ax) -> Add1/1
  oscilliation generator/2(Oscillation_ay) -> Add7/2
  oscilliation generator/3(Oscillation_az) -> Add5/1
  FSM_prrEcsAlgoFlag/1(isrEcsAlgoOutputs) -> S-Function Builder/1
  [Trigg_a2] -> FSM_prrEcsAlgoFlag/1(EcsFlag)
  S-Function Builder/2 -> SAD/1(prrFsmProfile)
  Ground/1 -> Rate Transition22/1
  Rate Transition7/1 -> PrevSolenoidCurrent/1
  PWM_to_V/1 -> Solenoid Model/1(SolenoidVoltage)
  A_to_mA/1 -> Rate Transition7/1
  [Trigg_a2] -> Solenoid Model/2(eCS_Trigger)
  PrevSolenoidCurrent/1 -> SAD/2(sim_au16Current)
  SAD/1(pseSolenoidPWM) -> PWM_to_V/1
  eCS_prrEcsDiagRequest_b8DiagReq1/1(b8DiagReq) -> eCS/2(prrEcsDiagRequest)
  Demux/1 -> BusCreator/1  "s16Ax"
  Demux/2 -> BusCreator/2  "s16Ay"
  Saturation1/1 -> eCS Algo new2/2(Pulse Z), BusCreator/3  "s16Az"
  BusCreator/1 -> eCS/1(prrAccelMtrPerSecSqd)  "stAccelMtrPerSecSqd"
  eCS/1(psrEcsAlgoData) -> Bus Selector1/1
  Bus Selector1/1 -> Data Type Conversion/1  "<b8EcsFlag>"
  Bus Selector1/2 -> [Ball_a2]  "<u16BallPosition>"
  Data Type Conversion/1 -> [Trigg_a2]
  Solenoid Model/1(SolenoidCurrent) -> A_to_mA/1
  S-Function Builder/1 -> Terminator4/1
  FSM_prrVehicleInputs/1(isrVehicleInputs) -> Terminator1/1
  eCS_prrAccelMtrPerSecSqd_stAccelMtrPerSecSqd/1(stAccelMtrPerSecSqd) -> Subsystem/1(prrAccelMtrPerSecSqd)
  eCS_prrEcsDiagRequest/1(isrEcsDiagRequest) -> Subsystem/2(prrEcsDiagRequest)

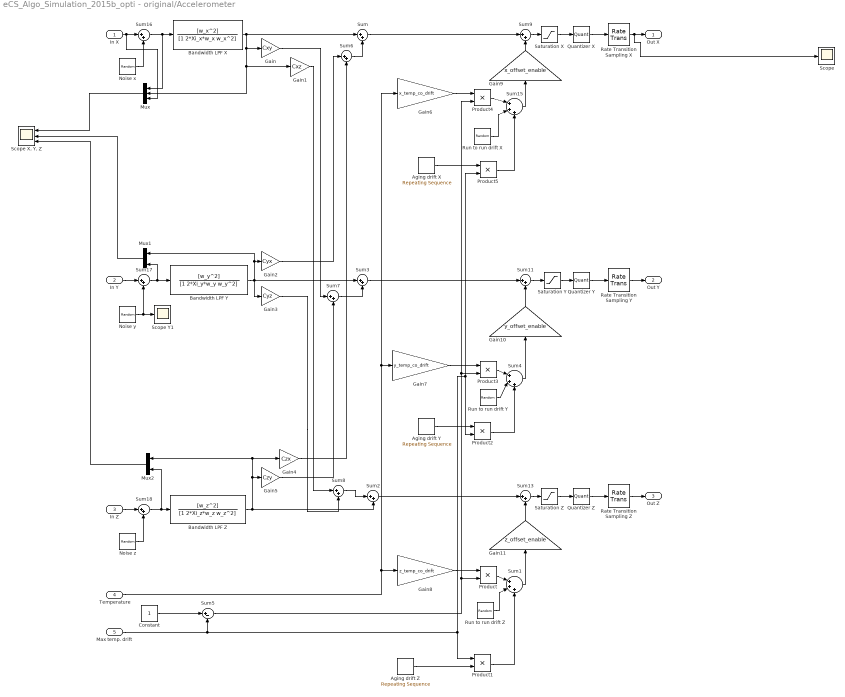
== system eCS_Algo_Simulation_2015b_opti - original/Accelerometer ==
  In X : Inport
  In Y : Inport  Port=2
  In Z : Inport  Port=3
  Temperature : Inport  Port=4
  Max temp. drift : Inport  Port=5
  Aging drift X : simulink/Sources/Repeating Sequence  rep_seq_t=[0 0.1]  rep_seq_y=[0 x_max_temp_drift]
  Aging drift Y : simulink/Sources/Repeating Sequence  rep_seq_t=[0 1000]  rep_seq_y=[0 y_max_temp_drift]
  Aging drift Z : simulink/Sources/Repeating Sequence  rep_seq_t=[0 0.001]  rep_seq_y=[0 z_max_temp_drift]
  Bandwidth LPF X : TransferFcn  Numerator=[w_x^2]  Denominator=[1 2*Xi_x*w_x w_x^2]
  Bandwidth LPF Y : TransferFcn  Numerator=[w_y^2]  Denominator=[1 2*Xi_y*w_y w_y^2]
  Bandwidth LPF Z : TransferFcn  Numerator=[w_z^2]  Denominator=[1 2*Xi_z*w_z w_z^2]
  Constant : Constant
  Gain : Gain  Gain=Cxy
  Gain1 : Gain  Gain=Cxz
  Gain10 : Gain  Gain=y_offset_enable
  Gain11 : Gain  Gain=z_offset_enable
  Gain2 : Gain  Gain=Cyx
  Gain3 : Gain  Gain=Cyz
  Gain4 : Gain  Gain=Czx
  Gain5 : Gain  Gain=Czy
  Gain6 : Gain  Gain=x_temp_co_drift
  Gain7 : Gain  Gain=y_temp_co_drift
  Gain8 : Gain  Gain=z_temp_co_drift
  Gain9 : Gain  Gain=x_offset_enable
  Mux : Mux  Inputs=3
  Mux1 : Mux  Inputs=2
  Mux2 : Mux  Inputs=2
  Noise x : RandomNumber  Mean=Mean_x_noise  Variance=Var_x_noise
  Noise y : RandomNumber  Mean=Mean_y_noise  Variance=Var_y_noise
  Noise z : RandomNumber  Mean=Mean_z_noise  Variance=Var_z_noise
  Product{,1..5} (6 alike) : Product  RndMeth=Zero
  Quantizer X : Quantizer  QuantizationInterval=Resolution
  Quantizer Y : Quantizer  QuantizationInterval=Resolution
  Quantizer Z : Quantizer  QuantizationInterval=Resolution
  Rate Transition Sampling X : RateTransition  OutPortSampleTime=1/ODR
  Rate Transition Sampling Y : RateTransition  OutPortSampleTime=1/ODR
  Rate Transition Sampling Z : RateTransition  OutPortSampleTime=1/ODR
  Run to run drift X : RandomNumber  Mean=x_run_to_run_drift  Variance=0.00001
  Run to run drift Y : RandomNumber  Mean=y_run_to_run_drift  Variance=0.00001
  Run to run drift Z : RandomNumber  Mean=z_run_to_run_drift  Variance=0.00001
  Saturation X : Saturate  UpperLimit=Range  LowerLimit=-Range
  Saturation Y : Saturate  UpperLimit=Range  LowerLimit=-Range
  Saturation Z : Saturate  UpperLimit=Range  LowerLimit=-Range
  Scope : Scope
  "Scope X, Y, Z" : Scope  NumInputPorts=3
  Scope Y1 : Scope
  Sum{,2..3,6..9,11,13,16..18} (12 alike) : Sum  Inputs=|++
  Sum1 : Sum  Inputs=|+++
  Sum15 : Sum  Inputs=|+++
  Sum4 : Sum  Inputs=|+++
  Sum5 : Sum  Inputs=|+-
  Out X : Outport
  Out Y : Outport  Port=2
  Out Z : Outport  Port=3
  wires:
  Run to run drift Z/1 -> Sum1/2
  Sum4/1 -> Gain10/1
  Run to run drift Y/1 -> Sum4/2
  Sum1/1 -> Gain11/1
  Bandwidth LPF Y/1 -> Gain3/1, Sum3/1, Mux1/1, Gain2/1
  Sum6/1 -> Sum/2
  Gain4/1 -> Sum6/2
  Bandwidth LPF Z/1 -> Mux2/1, Gain4/1, Gain5/1, Sum2/2
  Quantizer X/1 -> Rate Transition Sampling X/1
  Saturation Y/1 -> Quantizer Y/1
  Quantizer Z/1 -> Rate Transition Sampling Z/1
  Sum7/1 -> Sum3/2
  Gain5/1 -> Sum7/2
  Saturation X/1 -> Quantizer X/1
  Sum/1 -> Sum9/1
  Sum9/1 -> Saturation X/1
  Gain2/1 -> Sum6/1
  Sum3/1 -> Sum11/1
  Sum2/1 -> Sum13/1
  Sum13/1 -> Saturation Z/1
  Gain1/1 -> Sum8/1
  Run to run drift X/1 -> Sum15/2
  Gain3/1 -> Sum8/2
  Sum15/1 -> Gain9/1
  Sum11/1 -> Saturation Y/1
  In X/1 -> Mux/3, Sum16/1
  Sum16/1 -> Mux/1, Bandwidth LPF X/1
  Bandwidth LPF X/1 -> Mux/2, Gain1/1, Gain/1, Sum/1
  Gain/1 -> Sum7/1
  Quantizer Y/1 -> Rate Transition Sampling Y/1
  Saturation Z/1 -> Quantizer Z/1
  Noise z/1 -> Sum18/2
  Rate Transition Sampling Y/1 -> Out Y/1
  Sum17/1 -> Mux1/2, Bandwidth LPF Y/1
  Sum18/1 -> Bandwidth LPF Z/1, Mux2/2
  In Z/1 -> Sum18/1
  In Y/1 -> Sum17/1
  Rate Transition Sampling X/1 -> Scope/1, Out X/1
  Noise y/1 -> Scope Y1/1, Sum17/2
  Rate Transition Sampling Z/1 -> Out Z/1
  Noise x/1 -> Sum16/2
  Mux2/1 -> "Scope X, Y, Z"/3
  Temperature/1 -> Gain6/1, Gain7/1, Gain8/1
  Mux/1 -> "Scope X, Y, Z"/1
  Constant/1 -> Sum5/1
  Max temp. drift/1 -> Product2/2, Product5/2, Product1/1, Sum5/2
  Gain8/1 -> Product/1
  Product/1 -> Sum1/1
  Sum5/1 -> Product4/2, Product3/2, Product/2
  Product1/1 -> Sum1/3
  Aging drift Z/1 -> Product1/2
  Gain7/1 -> Product3/1
  Product3/1 -> Sum4/1
  Gain6/1 -> Product4/1
  Product4/1 -> Sum15/1
  Aging drift X/1 -> Product5/1
  Product5/1 -> Sum15/3
  Product2/1 -> Sum4/3
  Aging drift Y/1 -> Product2/1
  Sum8/1 -> Sum2/1
  Mux1/1 -> "Scope X, Y, Z"/2
  Gain9/1 -> Sum9/2
  Gain10/1 -> Sum11/2
  Gain11/1 -> Sum13/2

== system eCS_Algo_Simulation_2015b_opti - original/Crash signal1 ==
  Demux : Demux  Tag=STV Demux  Outputs=1
  FromWs : FromWorkspace  Tag=STV FromWs  VariableName=tuvar  SampleTime=0
      SigBuilderData=|
      | common.afterFinalStr = 'Extrapolate'
      | common.sampleTime = 0
      | dataSet.timeRange = [0 0.01]
      | dataSet.name = 'Group 1'
      | sbobj.Groups.Name = 'Group 1'
      | sbobj.Groups.Signals.Name = 'Signal 1'
      | sbobj.Groups.Signals.XData = [0 0.0005 0.001 0.001 0.0015 0.002 0.0025 0.00299 0.00299 0.0035 0.004 0.004 0.0045 0.0045 0.005 0.005 0.0055 0.0055 0.006 0.006 0.0065 0.007 0.007 0.0075 0.008 0.008 0.0085 0.009 0.0095 0.0095 0.01]
      | sbobj.Groups.Signals.YData = [0 2 2 1.99 2 2 2 2 0 0 0.015 0.02 0.005 0 2 2.005 3.96 3.98 6.04 6.03 6.02 6.04 6.06 6 5.98 0 -0.02 6 -0.02 0 0]
      | sbobj.Groups.TimeRange = [0 0.01]
  Signal 1 : Outport  Tag=STV Outport
  wires:
  Demux/1 -> Signal 1/1
  FromWs/1 -> Demux/1

== system eCS_Algo_Simulation_2015b_opti - original/Crash signal3 ==
  Demux : Demux  Tag=STV Demux  Outputs=1
  FromWs : FromWorkspace  Tag=STV FromWs  VariableName=tuvar  SampleTime=0
      SigBuilderData=|
      | common.afterFinalStr = 'Extrapolate'
      | common.sampleTime = 0
      | dataSet.timeRange = [0 0.01]
      | dataSet.name = 'Group 1'
      | sbobj.Groups.Name = 'Group 1'
      | sbobj.Groups.Signals.Name = 'Signal 1'
      | sbobj.Groups.Signals.XData = [0 0.0005 0.001 0.001 0.0015 0.002 0.0025 0.003 0.003 0.0035 0.004 0.004 0.0045 0.0045 0.005 0.005 0.0055 0.0055 0.006 0.006 0.0065 0.007 0.007 0.0075 0.008 0.008 0.0085 0.009 0.0095 0.0095 0.01]
      | sbobj.Groups.Signals.YData = [0 2 2 1.99 2 2 2 2 0 0 0.015 0.02 0.005 0 2 2.005 3.96 3.98 6.04 6.03 6.02 6.04 6.06 6 5.98 0 -0.02 6 -0.02 0 0]
      | sbobj.Groups.TimeRange = [0 0.01]
  Signal 1 : Outport  Tag=STV Outport
  wires:
  Demux/1 -> Signal 1/1
  FromWs/1 -> Demux/1

== system eCS_Algo_Simulation_2015b_opti - original/FSM ==
  prrEcsAlgoFlag : Inport
  Subsystem : Subsystem  Tag=struct('sfcnName','FSM_sf','subFunction','','srcSubsystem','')  mask(TL_Enable){}
      settings: OpenFcn=warndlg(get_param(gcb,'MaskHelp'),'Serious Warning');
      mask Help: This subsystem keeps the TargetLink subsystem (subsystem with TargetLink blocks for production code generation), and is needed for the TargetLink simulation frame to work properly. DO NOT DELETE OR MODIFY IT!
  psrSolenoidState : Outport
  psrFsmProfile : Outport  Port=2
  wires:
  prrEcsAlgoFlag/1 -> Subsystem/1(prrEcsAlgoFlag)
  Subsystem/1(psrSolenoidState) -> psrSolenoidState/1
  Subsystem/2(psrFsmProfile) -> psrFsmProfile/1

== system eCS_Algo_Simulation_2015b_opti - original/FSM_prrEcsAlgoFlag ==
  EcsFlag : Inport
  BusCreator : BusCreator  Inputs=2
  Const1 : Constant  Value=0
  isrEcsAlgoOutputs : Outport
  wires:
  EcsFlag/1 -> BusCreator/1  "b8EcsFlag"
  Const1/1 -> BusCreator/2  "u16BallPosition"
  BusCreator/1 -> isrEcsAlgoOutputs/1  "isrEcsAlgoOutputs"

== system eCS_Algo_Simulation_2015b_opti - original/FSM_prrVehicleInputs ==
  BusCreator : BusCreator  Inputs=2
  Const1 : Constant  Value=3
  Pulse measured1 : RateTransition  Deterministic=off  OutPortSampleTime=1/2000
  Ramp : simulink/Sources/Ramp  slope=1000  start=0  X0=0
  Scope : Scope
  isrVehicleInputs : Outport
  wires:
  Ramp/1 -> BusCreator/1, Scope/1  "u16Vx"
  Const1/1 -> BusCreator/2  "u8BuckleState"
  BusCreator/1 -> Pulse measured1/1  "isrVehicleInputs"
  Pulse measured1/1 -> isrVehicleInputs/1

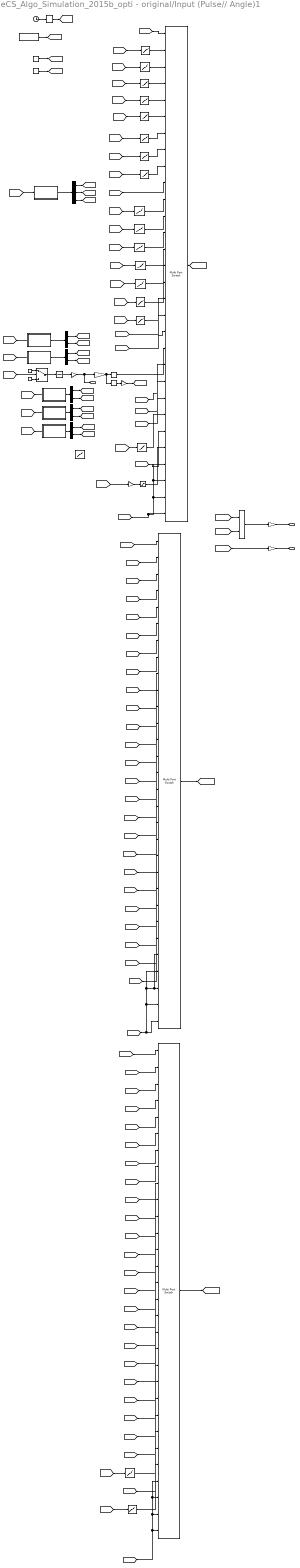
== system eCS_Algo_Simulation_2015b_opti - original/Input (Pulse// Angle)1 ==
  note: pulse tables must begin and end with 0 !!!!!!!
  -1.0 : Constant  Value=-1
  BMW QV72003-3 no-fire lower : Lookup_n-D  NumberOfTableDimensions=1  BreakpointsForDimension1=[-0.011 0.00 0.020 0.045 0.059]  Table=[0 0 11.0 11.0 0]  ExtrapMethod=Clip  UseLastTableValue=on  InternalRulePriority=Speed  RndMeth=Simplest  InputSameDT=on
  BMW QV72003-3 no-fire upper : Lookup_n-D  NumberOfTableDimensions=1  BreakpointsForDimension1=[0 0.027 0.059 0.085]  Table=[0 16.2 16.2 0]  ExtrapMethod=Clip  UseLastTableValue=on  InternalRulePriority=Speed  RndMeth=Simplest  InputSameDT=on
  Clock : Clock
  Demux1 : Demux  Outputs=3
  Demux{2..6} (5 alike) : Demux  Outputs=2
  Discrete-Time Integrator4 : DiscreteIntegrator  gainval=1  InitialConditionSetting=State (most efficient)  SampleTime=-1  UpperSaturationLimit=0.3 * 9.81  LowerSaturationLimit=-0.3 * 9.81  ICPrevOutput=DiscIntNeverNeededParam  ICPrevScaledInput=DiscIntNeverNeededParam
  Gain : Gain  Gain=-1
  Multiport Switch1 : MultiPortSwitch  Inputs=28  DataPortForDefault=Additional data port
  Multiport Switch2 : MultiPortSwitch  Inputs=28  DataPortForDefault=Additional data port
  Multiport Switch3 : MultiPortSwitch  Inputs=28  DataPortForDefault=Additional data port
  Mux1 : Mux  Inputs=2
  Puls_BMW_KSF_50 : Subsystem
  Puls_BMW_KSG_30 : Subsystem
  "Puls_BMW_Rauasphalt_60 " : Subsystem
  Puls_GWM_road_C.Morgan : Subsystem
  Puls_Kopfsteinpflaster Meldorf Hindenburgstrasse : Subsystem
  Puls_VW416_Atlas_C.Morgan : Subsystem
  Pulse table FF27 (g) : Lookup  InputValues=pulsetime_FF27  Table=pulse_FF27  LookUpMeth=Interpolation-Use End Values
  Pulse table MPDB (g) : Lookup  InputValues=pulsetime_MPDB  Table=pulse_MPDB  LookUpMeth=Interpolation-Use End Values
  Pulse table ODB40 (g) : Lookup  InputValues=pulsetime_ODB40  Table=pulse_ODB40  LookUpMeth=Interpolation-Use End Values
  Pulse table ODB64 (g) : Lookup  InputValues=pulsetime_ODB64  Table=pulse_ODB64  LookUpMeth=Interpolation-Use End Values
  Pulse table USNCAP (g) : Lookup  InputValues=pulsetime_USNCAP  Table=pulse_USNCAP  LookUpMeth=Interpolation-Use End Values
  Rate Transition : RateTransition
  Saturation : Saturate  UpperLimit=5  LowerLimit=0
  Sin1 : Trigonometry  Operator=cos
  Sin2 : Trigonometry
  Switch : Switch  Criteria=u2 > Threshold  Threshold=36
  crash angle in rad : Gain  Gain=2*pi/360
  g in m/s² : Gain  Gain=9.807
  g in m/s²1 : Gain  Gain=9.807
  "g-lock \" must lock\" - 6g/s - 0.45g" : Lookup_n-D  NumberOfTableDimensions=1  BreakpointsForDimension1=[0 0.075 0.3 0.4]  Table=[0 0.45 0.45 0]  ExtrapMethod=Clip  UseLastTableValue=on  InternalRulePriority=Speed  RndMeth=Simplest  InputSameDT=on
  "g-lock \" no lock\" - 6g/s - 0.3g" : Lookup_n-D  NumberOfTableDimensions=1  BreakpointsForDimension1=[0 0.050 0.5 0.6]  Table=[0 0.3 0.3 0]  ExtrapMethod=Clip  UseLastTableValue=on  InternalRulePriority=Speed  RndMeth=Simplest  InputSameDT=on
  g-lock Crash - 2000g/s - 30g : Lookup_n-D  NumberOfTableDimensions=1  BreakpointsForDimension1=[0 0.015 0.055 0.08]  Table=[0 30 30 0]  ExtrapMethod=Clip  UseLastTableValue=on  InternalRulePriority=Speed  RndMeth=Simplest  InputSameDT=on
  g-lock ECE - 150g/s - 0.45g : Lookup_n-D  NumberOfTableDimensions=1  BreakpointsForDimension1=[0 0.003 0.3 0.4]  Table=[0 0.45 0.45 0]  ExtrapMethod=Clip  UseLastTableValue=on  InternalRulePriority=Speed  RndMeth=Simplest  InputSameDT=on
  g-lock ECE - 25g/s - 0.45g : Lookup_n-D  NumberOfTableDimensions=1  BreakpointsForDimension1=[0 0.018 0.3 0.4]  Table=[0 0.45 0.45 0]  ExtrapMethod=Clip  UseLastTableValue=on  InternalRulePriority=Speed  RndMeth=Simplest  InputSameDT=on
  g-lock ECE - 25g/s - 0.45g custom : Lookup_n-D  NumberOfTableDimensions=1  BreakpointsForDimension1=[0 0.1 0.10001 1]  Table=[0 0 1 1]  ExtrapMethod=Clip  UseLastTableValue=on  InternalRulePriority=Speed  RndMeth=Simplest  InputSameDT=on
  g-lock ECE - 25g/s - 0.45g custom1 : Lookup_n-D  NumberOfTableDimensions=1  BreakpointsForDimension1=[0,0.018,0.3,0.4,0.6,0.618,1,1.1,3,3.018,3.05,3.1,3.118,3.5,3.6,4,4.018,4.2,4.3,8,8.018,8.1,8.15,9,9.018,9.3,9.4,10]  Table=[0,0.45,0.45,0,0,0.45,0.45,0,0,0.45,0.45,0,0.45,0.45,0,0,0.45,0.45,0,0,0.45,0.45,0,0,0.45,0.45,0,0]  ExtrapMethod=Clip  UseLastTableValue=on  InternalRulePriority=Speed  RndMeth=Simplest  InputSameDT=on
  g-lock FMVSS  - 16g/s - 0,7g : Lookup_n-D  NumberOfTableDimensions=1  BreakpointsForDimension1=[0 0.04375 0.3 0.4]  Table=[0 0.7 0.7 0]  ExtrapMethod=Clip  UseLastTableValue=on  InternalRulePriority=Speed  RndMeth=Simplest  InputSameDT=on
  g-lock FMVSS - 70g/s - 0.7g : Lookup_n-D  NumberOfTableDimensions=1  BreakpointsForDimension1=[0 0.01 0.3 0.4]  Table=[0 0.7 0.7 0]  ExtrapMethod=Clip  UseLastTableValue=on  InternalRulePriority=Speed  RndMeth=Simplest  InputSameDT=on
  g-lock Vollbremsung - 4g/s - 1g : Lookup_n-D  NumberOfTableDimensions=1  BreakpointsForDimension1=[0 0.25 0.9745 1.2]  Table=[0 1 1 0]  ExtrapMethod=Clip  UseLastTableValue=on  InternalRulePriority=Speed  RndMeth=Simplest  InputSameDT=on
  g_rate : Gain  Gain=5
  generic rollover : Lookup_n-D  NumberOfTableDimensions=1  BreakpointsForDimension1=[0 15 16 20 25 30 30.001 32 35 60]  Table=[-1 -1 1 1 0.5 0.5 0.49 0.49 -1 -1]  ExtrapMethod=Clip  UseLastTableValue=on  InternalRulePriority=Speed  RndMeth=Simplest  InputSameDT=on
  pulsetype : Constant  Value=pulsetype
  rollover ? : Lookup_n-D  NumberOfTableDimensions=1  BreakpointsForDimension1=[0 0.01 0.39 0.4]  Table=[0 1 1 0]  ExtrapMethod=Clip  UseLastTableValue=on  InternalRulePriority=Speed  RndMeth=Simplest  InputSameDT=on
  tilt speed : Gain  Gain=10
  time_const : Constant  Value=-1
  time_const1 : Constant
  zero : Constant  Value=0.0
  "Pulse_profile " : Outport
  Pulse z-axis : Outport  Port=2
  angle in ° : Outport  Port=3
  wires:
  crash angle in rad/1 -> Sin1/1, Sin2/1
  tilt speed/1 -> angle in °/1, crash angle in rad/1
  time_const1/1 -> Switch/3
  time_const/1 -> Switch/1
  Switch/1 -> Discrete-Time Integrator4/1
  Discrete-Time Integrator4/1 -> tilt speed/1
  g_rate/1 -> Saturation/1
  Mux1/1 -> g in m/s²/1
  g in m/s²/1 -> "Pulse_profile "/1
  Clock/1 -> Rate Transition/1
  [time] -> g-lock ECE - 150g/s - 0.45g/1
  [time] -> g-lock ECE - 25g/s - 0.45g/1
  [time] -> g-lock FMVSS  - 16g/s - 0,7g/1
  Rate Transition/1 -> [time]
  [time] -> g-lock FMVSS - 70g/s - 0.7g/1
  [time] -> "g-lock \" no lock\" - 6g/s - 0.3g"/1
  [time] -> "g-lock \" must lock\" - 6g/s - 0.45g"/1
  [time] -> g-lock Vollbremsung - 4g/s - 1g/1
  [time] -> g-lock Crash - 2000g/s - 30g/1
  [time] -> Pulse table USNCAP (g)/1
  [time] -> Switch/2
  [time] -> g_rate/1
  [time] -> Puls_Kopfsteinpflaster Meldorf Hindenburgstrasse/1(time in)
  pulsetype/1 -> [pulsetype]
  [pulsetype] -> Multiport Switch3/1
  [pulsetype] -> Multiport Switch2/1
  Puls_Kopfsteinpflaster Meldorf Hindenburgstrasse/1(pulse out [x,y] (g)) -> Demux1/1
  Demux1/1 -> [x_09]
  Demux1/2 -> [y_09]
  zero/1 -> [zero]
  [zero] -> Multiport Switch2/2
  [zero] -> Multiport Switch2/3
  [zero] -> Multiport Switch2/4
  [zero] -> Multiport Switch2/5
  [zero] -> Multiport Switch2/6
  [zero] -> Multiport Switch2/7
  [zero] -> Multiport Switch2/8
  [zero] -> Multiport Switch2/9
  [zero] -> Multiport Switch2/12
  [zero] -> Multiport Switch2/13
  [zero] -> Multiport Switch2/14
  [y_09] -> Multiport Switch2/10
  [zero] -> Multiport Switch2/11
  [y_17] -> Multiport Switch2/18
  [zero] -> Multiport Switch2/17
  [zero] -> Multiport Switch2/16
  [zero] -> Multiport Switch2/15
  [y_18] -> Multiport Switch2/19
  [zero] -> Multiport Switch2/20
  [time] -> Pulse table FF27 (g)/1
  [time] -> Pulse table ODB40 (g)/1
  [time] -> Pulse table ODB64 (g)/1
  [time] -> Pulse table MPDB (g)/1
  [time] -> BMW QV72003-3 no-fire upper/1
  [time] -> BMW QV72003-3 no-fire lower/1
  Demux2/2 -> [y_17]
  Demux2/1 -> [x_17]
  Puls_GWM_road_C.Morgan/1(pulse out [x,y] (g)) -> Demux2/1
  [time] -> Puls_GWM_road_C.Morgan/1(time in)
  Puls_VW416_Atlas_C.Morgan/1(pulse out [x,y] (g)) -> Demux3/1
  Demux3/1 -> [x_18]
  Demux3/2 -> [y_18]
  [time] -> Puls_VW416_Atlas_C.Morgan/1(time in)
  Saturation/1 -> Multiport Switch3/26
  g-lock ECE - 25g/s - 0.45g/1 -> Multiport Switch3/3
  g-lock FMVSS  - 16g/s - 0,7g/1 -> Multiport Switch3/4
  g-lock ECE - 150g/s - 0.45g/1 -> Multiport Switch3/2
  g-lock FMVSS - 70g/s - 0.7g/1 -> Multiport Switch3/5
  "g-lock \" no lock\" - 6g/s - 0.3g"/1 -> Multiport Switch3/6
  "g-lock \" must lock\" - 6g/s - 0.45g"/1 -> Multiport Switch3/7
  g-lock Vollbremsung - 4g/s - 1g/1 -> Multiport Switch3/8
  g-lock Crash - 2000g/s - 30g/1 -> Multiport Switch3/9
  [x_09] -> Multiport Switch3/10
  Pulse table USNCAP (g)/1 -> Multiport Switch3/11
  Pulse table FF27 (g)/1 -> Multiport Switch3/12
  Pulse table ODB40 (g)/1 -> Multiport Switch3/13
  Pulse table ODB64 (g)/1 -> Multiport Switch3/14
  Pulse table MPDB (g)/1 -> Multiport Switch3/15
  BMW QV72003-3 no-fire upper/1 -> Multiport Switch3/16
  BMW QV72003-3 no-fire lower/1 -> Multiport Switch3/17
  [x_17] -> Multiport Switch3/18
  [x_18] -> Multiport Switch3/19
  Sin2/1 -> Multiport Switch3/20
  [zero] -> Multiport Switch2/25
  [y_09] -> Multiport Switch2/24
  [y_20] -> Multiport Switch2/21
  [y_21] -> Multiport Switch2/22
  [y_22] -> Multiport Switch2/23
  [x_20] -> Multiport Switch3/21
  [x_22] -> Multiport Switch3/23
  [x_21] -> Multiport Switch3/22
  Puls_BMW_KSF_50/1(pulse out [x,y] (g)) -> Demux4/1
  [time] -> Puls_BMW_KSF_50/1(time in)
  Demux4/1 -> [x_20]
  Demux4/2 -> [y_20]
  [time] -> Puls_BMW_KSG_30/1(time in)
  Puls_BMW_KSG_30/1(pulse out [x,y] (g)) -> Demux5/1
  Demux5/1 -> [x_21]
  Demux5/2 -> [y_21]
  "Puls_BMW_Rauasphalt_60 "/1(pulse out [x,y] (g)) -> Demux6/1
  [time] -> "Puls_BMW_Rauasphalt_60 "/1(time in)
  Demux6/1 -> [x_22]
  Demux6/2 -> [y_22]
  [minus_one] -> Multiport Switch1/23
  [minus_one] -> Multiport Switch1/22
  [minus_one] -> Multiport Switch1/21
  generic rollover/1 -> Multiport Switch1/24
  [minus_one] -> Multiport Switch1/25
  rollover ?/1 -> Multiport Switch1/26
  [z_19] -> Multiport Switch1/20
  [minus_one] -> Multiport Switch1/19
  [minus_one] -> Multiport Switch1/15
  [minus_one] -> Multiport Switch1/16
  [minus_one] -> Multiport Switch1/17
  [minus_one] -> Multiport Switch1/18
  [minus_one] -> Multiport Switch1/11
  [z_09] -> Multiport Switch1/10
  [minus_one] -> Multiport Switch1/14
  [minus_one] -> Multiport Switch1/13
  [minus_one] -> Multiport Switch1/12
  [minus_one] -> Multiport Switch1/9
  [minus_one] -> Multiport Switch1/8
  [minus_one] -> Multiport Switch1/7
  [minus_one] -> Multiport Switch1/6
  [minus_one] -> Multiport Switch1/5
  [minus_one] -> Multiport Switch1/4
  [minus_one] -> Multiport Switch1/3
  [minus_one] -> Multiport Switch1/2
  [pulsetype] -> Multiport Switch1/1
  Multiport Switch1/1 -> [z_acceleration]
  Multiport Switch2/1 -> [y_acceleration]
  [y_acceleration] -> Mux1/2  "ay(g)"
  [x_acceleration] -> Mux1/1  "ax(g)"
  Multiport Switch3/1 -> [x_acceleration]
  [z_acceleration] -> g in m/s²1/1  "az(g)"
  [time] -> rollover ?/1
  -1.0/1 -> [minus_one]
  g in m/s²1/1 -> Pulse z-axis/1
  Demux1/3 -> [z_09]
  Sin1/1 -> Gain/1
  Gain/1 -> [z_19]
  [time] -> generic rollover/1
  [x_09] -> Multiport Switch3/25
  [zero] -> Multiport Switch3/27, Multiport Switch3/28, Multiport Switch3/29, Multiport Switch3/30
  [zero] -> Multiport Switch2/27, Multiport Switch2/26, Multiport Switch2/28, Multiport Switch2/29, Multiport Switch2/30
  [minus_one] -> Multiport Switch1/27, Multiport Switch1/28, Multiport Switch1/29, Multiport Switch1/30
  [time] -> g-lock ECE - 25g/s - 0.45g custom/1
  g-lock ECE - 25g/s - 0.45g custom/1 -> Multiport Switch3/24

== system eCS_Algo_Simulation_2015b_opti - original/Noisy ==
  Demux : Demux  Tag=STV Demux  Outputs=1
  FromWs : FromWorkspace  Tag=STV FromWs  VariableName=tuvar  SampleTime=0
      SigBuilderData=|
      | common.afterFinalStr = 'Extrapolate'
      | common.sampleTime = 0
      | dataSet.timeRange = [0 0.01]
      | dataSet.name = 'Group 1'
      | sbobj.Groups.Name = 'Group 1'
      | sbobj.Groups.Signals.Name = 'Signal 1'
      | sbobj.Groups.Signals.XData = [0 0.0005 0.001 0.001 0.0015 0.0015 0.002 0.002 0.0025 0.0025 0.003 0.003 0.0035 0.0035 0.004 0.004 0.0045 0.0045 0.005 0.005 0.0055 0.0055 0.006 0.006 0.0065 0.007 0.007 0.0075 0.0075 0.008 0.008 0.0085 0.009 0.0095 0.0095 0.01]
      | sbobj.Groups.Signals.YData = [0 0 1.26 0.79 0.8 0.02 0.02 1.11 1.11 0.8 0.8 0 0 -0.02 1 0.02 0.005 0 0.63 0.65 0.9 0.22 1.09 0.04 0.4 1.58 1.18 1.12 0.32 0.8 0 -0.02 1.12 -0.02 0 0]
      | sbobj.Groups.TimeRange = [0 0.01]
  Signal 1 : Outport  Tag=STV Outport
  wires:
  FromWs/1 -> Demux/1
  Demux/1 -> Signal 1/1
